simulink model "btMuxTest"  (R2015b)
settings: Solver=FixedStepDiscrete  StartTime=0.0  StopTime=Inf  RelTol=1e-3
libraries: sensorLibrary x2, freescalecupcompanionlib x1, bluetoothLibrary x1
settings Model: SimulationMode=external  ExtModeTrigDuration=5  Creator=dc315  LastModifiedBy=dc315
settings OptimizationCC: OptimizeModelRefInitCode=on  LifeSpan=1  MaxStackSize=64
settings HardwareCC: ProdBitPerPointer=32  ProdLargestAtomicInteger=Long  ProdLargestAtomicFloat=Double  ProdWordSize=32  ProdHWDeviceType=ARM Compatible->ARM Cortex
settings RTWCC: SystemTargetFile=ert.tlc  TemplateMakefile=ert_default_tmf  Description=Embedded Coder  Toolchain=GNU Tools for ARM Embedded Processors
settings CodeAppCC: IgnoreCustomStorageClasses=off

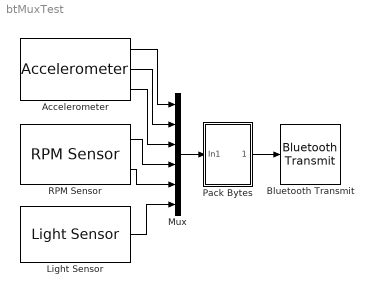
== system btMuxTest ==
  Accelerometer : freescalecupcompanionlib/Accelerometer  SampleTime=0.01
  Bluetooth Transmit : bluetoothLibrary/Bluetooth Transmit  baudRate=9600
  Light Sensor : sensorLibrary/Light Sensor  Gain=20
  Mux : Mux  Inputs=6
  Pack Bytes : Subsystem  mask{Value=77554433}
      mask prompts: Value "Header"
      mask TypeOptions Value: Constant/Value
      mask Display:
      | pic = imread('pack_icon.jpg');
      | image(pic,'center');
  RPM Sensor : sensorLibrary/RPM Sensor  SystemSampleTime=-1
  wires:
  Accelerometer/1 -> Mux/1
  Accelerometer/2 -> Mux/2
  Accelerometer/3 -> Mux/3
  Mux/1 -> Pack Bytes/1(In1)
  Pack Bytes/1(Out1) -> Bluetooth Transmit/1
  Light Sensor/1 -> Mux/6
  RPM Sensor/2 -> Mux/5
  RPM Sensor/1 -> Mux/4

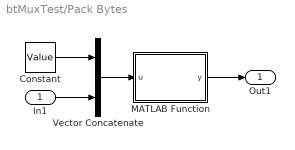
== system btMuxTest/Pack Bytes ==
  In1 : Inport
  Constant : Constant  Value=Value
  MATLAB Function : MATLAB Function  TreatAsAtomicUnit=on
  Vector Concatenate : Concatenate
  Out1 : Outport
  wires:
  In1/1 -> Vector Concatenate/2
  MATLAB Function/1(y) -> Out1/1
  Constant/1 -> Vector Concatenate/1
  Vector Concatenate/1 -> MATLAB Function/1(u)

== matlab function btMuxTest/Pack Bytes/MATLAB Function ==
  data: u input; y output
function y = fcn(u)
%#codegen

y = typecast(u,'uint8');
